simulink model "source"  (R2014b)
settings: Solver=ode23tb  StartTime=0.0  StopTime=5  MaxStep=.00001  RelTol=1e-3
libraries: powerlib x54
settings Model: Creator=Muruganandham AP  LastModifiedBy=SELVA
settings SolverCC: ZeroCrossControl=DisableAll
settings DataIOCC: SignalLoggingSaveFormat=ModelDataLogs
settings OptimizationCC: ExpressionDepthLimit=2147483647
settings DebuggingCC: UnderspecifiedInitializationDetection=Classic  MergeDetectMultiDrivingBlocksExec=none  FcnCallInpInsideContextMsg=UseLocalSettings  StateNameClashWarn=warning
settings GRTTargetCC: CombineOutputUpdateFcns=off  GRTInterface=on

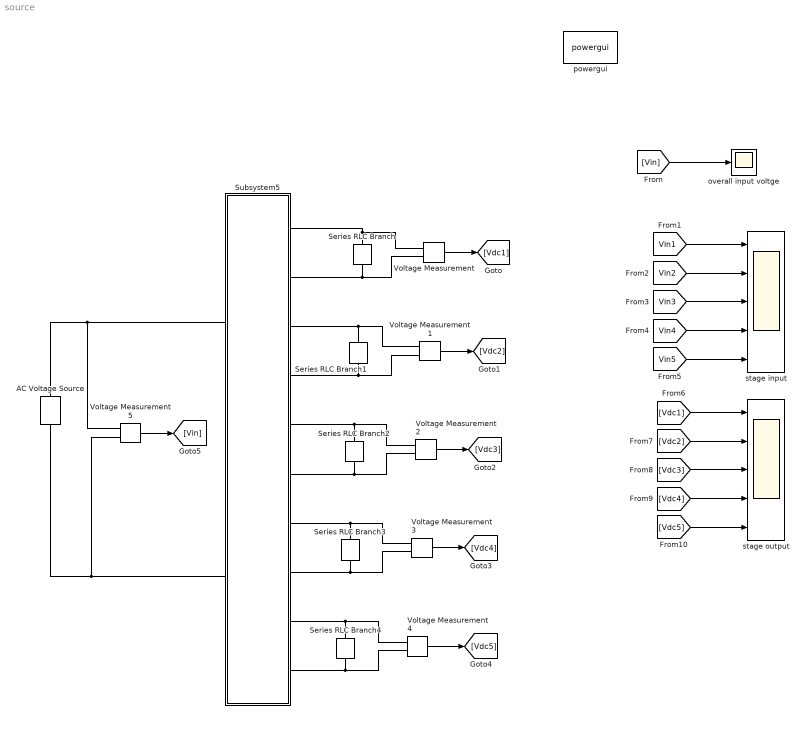
== system source ==
  AC Voltage Source : powerlib/Electrical Sources/AC Voltage Source  Amplitude=230*sqrt(2)  Phase=0  Frequency=50  SampleTime=0  Measurements=None
  Series RLC Branch{,1..4} (5 alike) : powerlib/Elements/Series RLC Branch  LConnTagsString=__new0  RConnTagsString=__new0  BranchType=R  Resistance=100  Inductance=1e-3  SetiL0=off  InitialCurrent=0  Capacitance=1e-6  Setx0=off  InitialVoltage=0  Measurements=None
  Subsystem5 : Subsystem
  Voltage Measurement{,1..5} (6 alike) : powerlib/Measurements/Voltage Measurement  PhasorSimulation=off  OutputType=Complex  PSBequivalent=0
  "overall input voltge " : Scope
  powergui : powerlib/powergui  Priority=1  SimulationMode=Discrete  SolverType=Tustin/Backward Euler (TBE)  SampleTime=50e-6  frequency=60  SPID=off  DisableSnubberDevices=off  DisableRonSwitches=off  DisableVfSwitches=off  SwTol=0  DisplayEquations=off  Interpol=off  methode=off  Ts=100  frequencyindice=50  Pbase=100e6  ErrMax=1e-4  Iterations=50  UnitsV=kV  UnitsW=MW  FunctionMessages=off  echomessages=off  HookPort=off  EnableUseOfTLC=off  x0status=blocks  RestoreLinks=warning  ResistiveCurrentMeasurement=off  Frange=[0:2:500]  Ylog=off  Xlog=on  ShowGrid=off  save=off  variable=ZData  structure=0  ZoomFFT=off  StartTime=0.0  cycles=1  DisplayStyle=1  fundamental=60  FreqAxis=off  MaxFrequency=1000  frequencyindicesteady=1  RmsSteady=1  display=off
  stage input : Scope  NumInputPorts=5
      settings: YMin=-5~-5~-5~-5~-5  YMax=5~5~5~5~5  SaveName=ScopeData2
  stage output : Scope  NumInputPorts=5
      settings: YMin=-5~-5~-5~-5~-5  YMax=5~5~5~5~5  SaveName=ScopeData3
  wires:
  Voltage Measurement/1 -> [Vdc1]
  Voltage Measurement1/1 -> [Vdc2]
  Voltage Measurement2/1 -> [Vdc3]
  Voltage Measurement3/1 -> [Vdc4]
  Voltage Measurement4/1 -> [Vdc5]
  Voltage Measurement5/1 -> [Vin]
  [Vin] -> "overall input voltge "/1
  [Vin1] -> stage input/1
  [Vin2] -> stage input/2
  [Vin3] -> stage input/3
  [Vin4] -> stage input/4
  [Vin5] -> stage input/5
  [Vdc1] -> stage output/1
  [Vdc2] -> stage output/2
  [Vdc3] -> stage output/3
  [Vdc4] -> stage output/4
  [Vdc5] -> stage output/5
  connections:
  AC Voltage Source/RConn1 -- Subsystem5/LConn1 -- Voltage Measurement5/LConn1
  AC Voltage Source/LConn1 -- Subsystem5/LConn2 -- Voltage Measurement5/LConn2
  Subsystem5/RConn1 -- Series RLC Branch/LConn1 -- Voltage Measurement/LConn1
  Voltage Measurement1/LConn2 -- Subsystem5/RConn4 -- Series RLC Branch1/RConn1
  Subsystem5/RConn5 -- Series RLC Branch2/LConn1 -- Voltage Measurement2/LConn1
  Subsystem5/RConn6 -- Series RLC Branch2/RConn1 -- Voltage Measurement2/LConn2
  Subsystem5/RConn7 -- Voltage Measurement3/LConn1 -- Series RLC Branch3/LConn1
  Subsystem5/RConn8 -- Voltage Measurement3/LConn2 -- Series RLC Branch3/RConn1
  Subsystem5/RConn9 -- Series RLC Branch4/LConn1 -- Voltage Measurement4/LConn1
  Subsystem5/RConn10 -- Series RLC Branch4/RConn1 -- Voltage Measurement4/LConn2
  Subsystem5/RConn2 -- Series RLC Branch/RConn1 -- Voltage Measurement/LConn2
  Subsystem5/RConn3 -- Series RLC Branch1/LConn1 -- Voltage Measurement1/LConn1

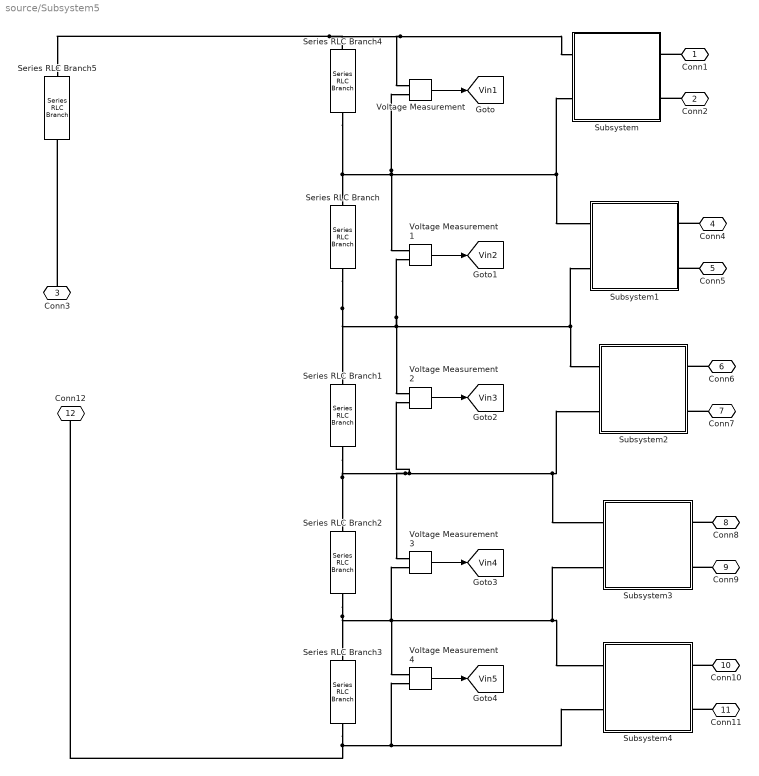
== system source/Subsystem5 ==
  Series RLC Branch{,1..4} (5 alike) : powerlib/Elements/Series RLC Branch  LConnTagsString=__new0  RConnTagsString=__new0  BranchType=C  Resistance=1  Inductance=1e-3  SetiL0=off  InitialCurrent=0  Capacitance=2500e-6  Setx0=off  InitialVoltage=0  Measurements=None
  Series RLC Branch5 : powerlib/Elements/Series RLC Branch  LConnTagsString=__new0  RConnTagsString=__new0  BranchType=R  Resistance=.001  Inductance=1e-3  SetiL0=off  InitialCurrent=0  Capacitance=2500e-6  Setx0=off  InitialVoltage=0  Measurements=None
  Subsystem : Subsystem
  Subsystem1 : Subsystem
  Subsystem2 : Subsystem
  Subsystem3 : Subsystem
  Subsystem4 : Subsystem
  Voltage Measurement{,1..4} (5 alike) : powerlib/Measurements/Voltage Measurement  PhasorSimulation=off  OutputType=Complex  PSBequivalent=0
  Conn1 : PMIOPort  Port=1  Side=Right
  Conn2 : PMIOPort  Port=2  Side=Right
  Conn3 : PMIOPort  Port=3  Side=Left
  Conn4 : PMIOPort  Port=4  Side=Right
  Conn5 : PMIOPort  Port=5  Side=Right
  Conn6 : PMIOPort  Port=6  Side=Right
  Conn7 : PMIOPort  Port=7  Side=Right
  Conn8 : PMIOPort  Port=8  Side=Right
  Conn9 : PMIOPort  Port=9  Side=Right
  Conn10 : PMIOPort  Port=10  Side=Right
  Conn11 : PMIOPort  Port=11  Side=Right
  Conn12 : PMIOPort  Port=12  Side=Left
  tag scope: Vin1=global, Vin2=global, Vin3=global, Vin4=global, Vin5=global
  wires:
  Voltage Measurement/1 -> [Vin1]
  Voltage Measurement1/1 -> [Vin2]
  Voltage Measurement2/1 -> [Vin3]
  Voltage Measurement3/1 -> [Vin4]
  Voltage Measurement4/1 -> [Vin5]
  connections:
  Series RLC Branch4/RConn1 -- Series RLC Branch/LConn1 -- Subsystem/LConn2 -- Subsystem1/LConn1 -- Voltage Measurement/LConn2 -- Voltage Measurement1/LConn1
  Series RLC Branch/RConn1 -- Series RLC Branch1/LConn1 -- Subsystem1/LConn2 -- Subsystem2/LConn1 -- Voltage Measurement1/LConn2 -- Voltage Measurement2/LConn1
  Series RLC Branch1/RConn1 -- Series RLC Branch2/LConn1 -- Subsystem2/LConn2 -- Subsystem3/LConn1 -- Voltage Measurement2/LConn2 -- Voltage Measurement3/LConn1
  Series RLC Branch2/RConn1 -- Series RLC Branch3/LConn1 -- Subsystem3/LConn2 -- Subsystem4/LConn1 -- Voltage Measurement3/LConn2 -- Voltage Measurement4/LConn1
  Series RLC Branch3/RConn1 -- Conn12/RConn1 -- Subsystem4/LConn2 -- Voltage Measurement4/LConn2
  Series RLC Branch4/LConn1 -- Series RLC Branch5/LConn1 -- Subsystem/LConn1 -- Voltage Measurement/LConn1
  Conn1/RConn1 -- Subsystem/RConn1
  Conn2/RConn1 -- Subsystem/RConn2
  Conn3/RConn1 -- Series RLC Branch5/RConn1
  Conn4/RConn1 -- Subsystem1/RConn1
  Conn5/RConn1 -- Subsystem1/RConn2
  Conn6/RConn1 -- Subsystem2/RConn1
  Conn7/RConn1 -- Subsystem2/RConn2
  Conn8/RConn1 -- Subsystem3/RConn1
  Conn9/RConn1 -- Subsystem3/RConn2
  Conn10/RConn1 -- Subsystem4/RConn1
  Conn11/RConn1 -- Subsystem4/RConn2

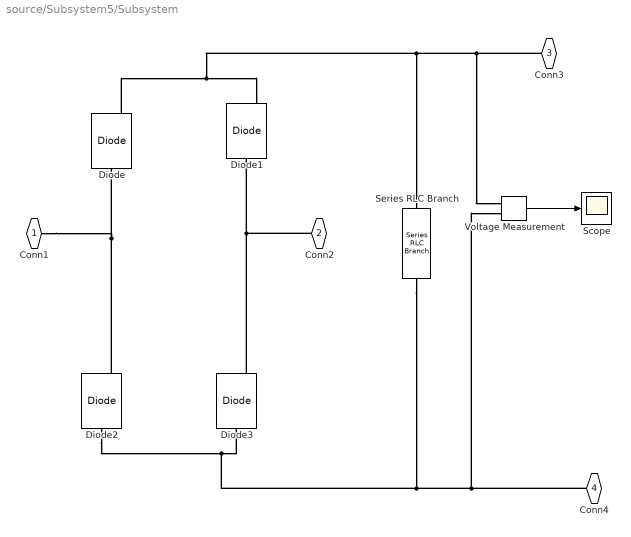
== system source/Subsystem5/Subsystem ==
  Diode{,1..3} (4 alike) : powerlib/Power Electronics/Diode  Ron=0.001  Lon=0  Vf=0.8  IC=0  UseSnubber=off  Rs=500  Cs=250e-9  Measurements=on
  Scope : Scope
      settings: TimeRange=1.601532567049809  YMin=9.312500000000002  YMax=11.5625
  Series RLC Branch : powerlib/Elements/Series RLC Branch  LConnTagsString=__new0  RConnTagsString=__new0  BranchType=C  Resistance=1  Inductance=1e-3  SetiL0=off  InitialCurrent=0  Capacitance=25000e-6  Setx0=off  InitialVoltage=0  Measurements=None
  Voltage Measurement : powerlib/Measurements/Voltage Measurement  PhasorSimulation=off  OutputType=Complex  PSBequivalent=0
  Conn1 : PMIOPort  Port=1  Side=Left
  Conn2 : PMIOPort  Port=2  Side=Left
  Conn3 : PMIOPort  Port=3  Side=Right
  Conn4 : PMIOPort  Port=4  Side=Right
  wires:
  Voltage Measurement/1 -> Scope/1
  connections:
  Conn4/RConn1 -- Voltage Measurement/LConn2 -- Diode2/LConn1 -- Diode3/LConn1 -- Series RLC Branch/RConn1
  Diode2/RConn1 -- Diode/LConn1 -- Conn1/RConn1
  Conn3/RConn1 -- Voltage Measurement/LConn1 -- Diode/RConn1 -- Diode1/RConn1 -- Series RLC Branch/LConn1
  Diode3/RConn1 -- Diode1/LConn1 -- Conn2/RConn1

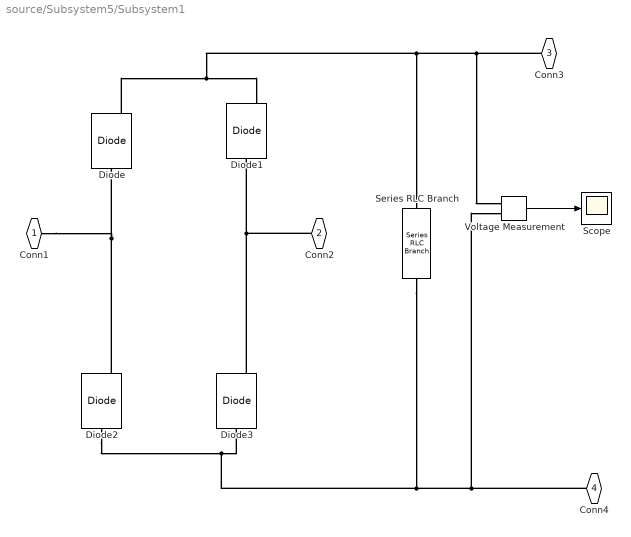
== system source/Subsystem5/Subsystem1 ==
  Diode{,1..3} (4 alike) : powerlib/Power Electronics/Diode  Ron=0.001  Lon=0  Vf=0.8  IC=0  UseSnubber=off  Rs=500  Cs=250e-9  Measurements=on
  Scope : Scope
      settings: TimeRange=1.601532567049809  YMin=9.312500000000002  YMax=11.5625
  Series RLC Branch : powerlib/Elements/Series RLC Branch  LConnTagsString=__new0  RConnTagsString=__new0  BranchType=C  Resistance=1  Inductance=1e-3  SetiL0=off  InitialCurrent=0  Capacitance=25000e-6  Setx0=off  InitialVoltage=0  Measurements=None
  Voltage Measurement : powerlib/Measurements/Voltage Measurement  PhasorSimulation=off  OutputType=Complex  PSBequivalent=0
  Conn1 : PMIOPort  Port=1  Side=Left
  Conn2 : PMIOPort  Port=2  Side=Left
  Conn3 : PMIOPort  Port=3  Side=Right
  Conn4 : PMIOPort  Port=4  Side=Right
  wires:
  Voltage Measurement/1 -> Scope/1
  connections:
  Conn2/RConn1 -- Diode1/LConn1 -- Diode3/RConn1
  Conn3/RConn1 -- Series RLC Branch/LConn1 -- Diode1/RConn1 -- Diode/RConn1 -- Voltage Measurement/LConn1
  Conn1/RConn1 -- Diode/LConn1 -- Diode2/RConn1
  Conn4/RConn1 -- Series RLC Branch/RConn1 -- Diode3/LConn1 -- Diode2/LConn1 -- Voltage Measurement/LConn2

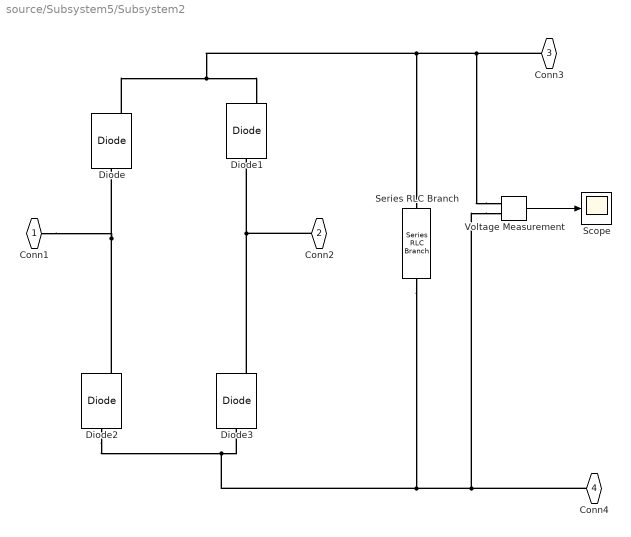
== system source/Subsystem5/Subsystem2 ==
  Diode{,1..3} (4 alike) : powerlib/Power Electronics/Diode  Ron=0.001  Lon=0  Vf=0.8  IC=0  UseSnubber=off  Rs=500  Cs=250e-9  Measurements=on
  Scope : Scope
      settings: TimeRange=1.601532567049809  YMin=9.312500000000002  YMax=11.5625
  Series RLC Branch : powerlib/Elements/Series RLC Branch  LConnTagsString=__new0  RConnTagsString=__new0  BranchType=C  Resistance=1  Inductance=1e-3  SetiL0=off  InitialCurrent=0  Capacitance=25000e-6  Setx0=off  InitialVoltage=0  Measurements=None
  Voltage Measurement : powerlib/Measurements/Voltage Measurement  PhasorSimulation=off  OutputType=Complex  PSBequivalent=0
  Conn1 : PMIOPort  Port=1  Side=Left
  Conn2 : PMIOPort  Port=2  Side=Left
  Conn3 : PMIOPort  Port=3  Side=Right
  Conn4 : PMIOPort  Port=4  Side=Right
  wires:
  Voltage Measurement/1 -> Scope/1
  connections:
  Voltage Measurement/LConn2 -- Diode2/LConn1 -- Diode3/LConn1 -- Series RLC Branch/RConn1 -- Conn4/RConn1
  Diode2/RConn1 -- Diode/LConn1 -- Conn1/RConn1
  Voltage Measurement/LConn1 -- Diode/RConn1 -- Diode1/RConn1 -- Series RLC Branch/LConn1 -- Conn3/RConn1
  Diode3/RConn1 -- Diode1/LConn1 -- Conn2/RConn1

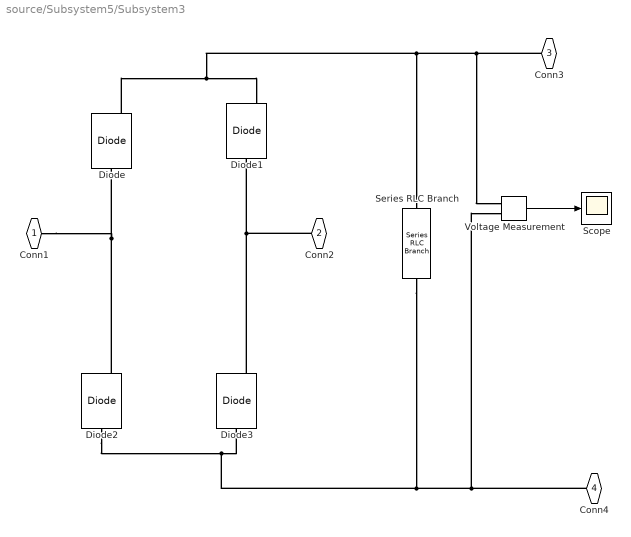
== system source/Subsystem5/Subsystem3 ==
  Diode{,1..3} (4 alike) : powerlib/Power Electronics/Diode  Ron=0.001  Lon=0  Vf=0.8  IC=0  UseSnubber=off  Rs=500  Cs=250e-9  Measurements=on
  Scope : Scope
      settings: TimeRange=1.601532567049809  YMin=9.312500000000002  YMax=11.5625
  Series RLC Branch : powerlib/Elements/Series RLC Branch  LConnTagsString=__new0  RConnTagsString=__new0  BranchType=C  Resistance=1  Inductance=1e-3  SetiL0=off  InitialCurrent=0  Capacitance=25000e-6  Setx0=off  InitialVoltage=0  Measurements=None
  Voltage Measurement : powerlib/Measurements/Voltage Measurement  PhasorSimulation=off  OutputType=Complex  PSBequivalent=0
  Conn1 : PMIOPort  Port=1  Side=Left
  Conn2 : PMIOPort  Port=2  Side=Left
  Conn3 : PMIOPort  Port=3  Side=Right
  Conn4 : PMIOPort  Port=4  Side=Right
  wires:
  Voltage Measurement/1 -> Scope/1
  connections:
  Conn2/RConn1 -- Diode1/LConn1 -- Diode3/RConn1
  Conn3/RConn1 -- Series RLC Branch/LConn1 -- Diode1/RConn1 -- Diode/RConn1 -- Voltage Measurement/LConn1
  Conn1/RConn1 -- Diode/LConn1 -- Diode2/RConn1
  Conn4/RConn1 -- Series RLC Branch/RConn1 -- Diode3/LConn1 -- Diode2/LConn1 -- Voltage Measurement/LConn2

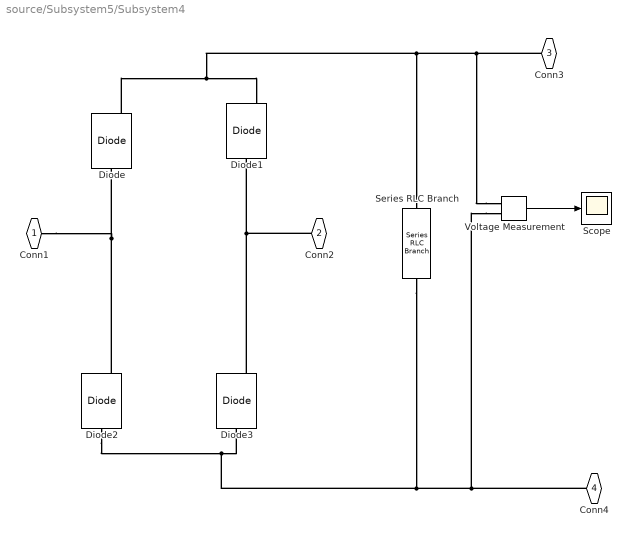
== system source/Subsystem5/Subsystem4 ==
  Diode{,1..3} (4 alike) : powerlib/Power Electronics/Diode  Ron=0.001  Lon=0  Vf=0.8  IC=0  UseSnubber=off  Rs=500  Cs=250e-9  Measurements=on
  Scope : Scope
      settings: TimeRange=1.601532567049809  YMin=9.312500000000002  YMax=11.5625
  Series RLC Branch : powerlib/Elements/Series RLC Branch  LConnTagsString=__new0  RConnTagsString=__new0  BranchType=C  Resistance=1  Inductance=1e-3  SetiL0=off  InitialCurrent=0  Capacitance=25000e-6  Setx0=off  InitialVoltage=0  Measurements=None
  Voltage Measurement : powerlib/Measurements/Voltage Measurement  PhasorSimulation=off  OutputType=Complex  PSBequivalent=0
  Conn1 : PMIOPort  Port=1  Side=Left
  Conn2 : PMIOPort  Port=2  Side=Left
  Conn3 : PMIOPort  Port=3  Side=Right
  Conn4 : PMIOPort  Port=4  Side=Right
  wires:
  Voltage Measurement/1 -> Scope/1
  connections:
  Voltage Measurement/LConn2 -- Diode2/LConn1 -- Diode3/LConn1 -- Series RLC Branch/RConn1 -- Conn4/RConn1
  Diode2/RConn1 -- Diode/LConn1 -- Conn1/RConn1
  Voltage Measurement/LConn1 -- Diode/RConn1 -- Diode1/RConn1 -- Series RLC Branch/LConn1 -- Conn3/RConn1
  Diode3/RConn1 -- Diode1/LConn1 -- Conn2/RConn1
